simulink model "StateSpaceDynamic"  (R2018a)
settings: Solver=VariableStepAuto  StartTime=0.0  StopTime=10.0  RelTol=1e-3
model workspace (MAT data in the model file):
  Iz = 0.05807429185
  cf = 50000
  cr = 50000
  k1 = 1
  k2 = 0.5673
  k3 = 2.6383
  k4 = 0.4975
  lf = 0.16002
  lr = 0.16002
  m = 2.26796
libraries: cstblocks x1
settings Model: Creator=aswer  LastModifiedBy=aswer

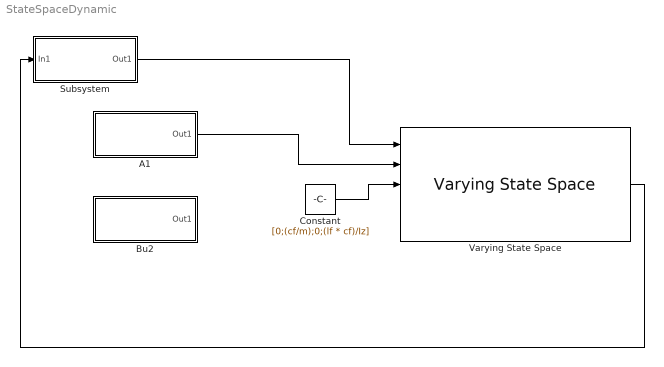
== system StateSpaceDynamic ==
  A1 : Subsystem
  Bu2 : Subsystem
  Constant : Constant  Value=[0;(cf/m);0;(lf * cf)/Iz]  VectorParams1D=off
  Subsystem : Subsystem
  Varying State Space : cstblocks/Linear Parameter Varying/Varying State Space  x0=0  xNames=''  OutputX=on  OutputDX=on
      settings: SourceProductName=Control System Toolbox
  wires:
  Varying State Space/2 -> Subsystem/1(In1)
  A1/1(Out1) -> Varying State Space/2
  Constant/1 -> Varying State Space/3
  Subsystem/1(Out1) -> Varying State Space/1

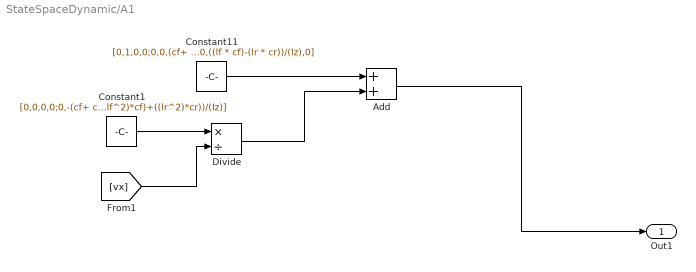
== system StateSpaceDynamic/A1 ==
  Add : Sum
  Constant1 : Constant  Value=[0,0,0,0;0,-(cf+ cr)/(m),0,(lr * cr)-(lf * cf)/(m);0,0,0,0;0,((lr * cr)-(lf * cf))/(Iz),0,-(((lf^2)*cf)+((lr^2)*cr))/(Iz)]  VectorParams1D=off
  Constant11 : Constant  Value=[0,1,0,0;0,0,(cf+ cr)/(m),0;0,0,0,1;0,0,((lf * cf)-(lr * cr))/(Iz),0]  VectorParams1D=off
  Divide : Product  Inputs=*/
  Out1 : Outport
  wires:
  [vx] -> Divide/2
  Constant11/1 -> Add/1
  Constant1/1 -> Divide/1
  Divide/1 -> Add/2
  Add/1 -> Out1/1

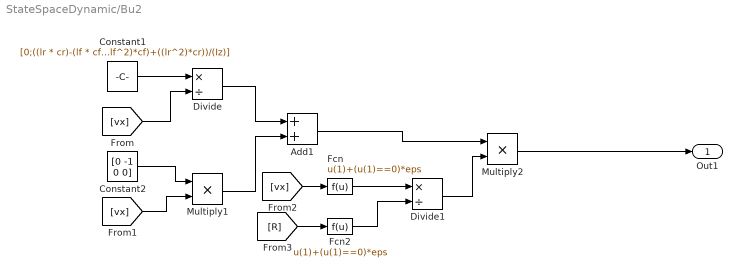
== system StateSpaceDynamic/Bu2 ==
  Add1 : Sum
  Constant1 : Constant  Value=[0;((lr * cr)-(lf * cf))/m;0;-(((lf^2)*cf)+((lr^2)*cr))/(Iz)]  VectorParams1D=off
  Constant2 : Constant  Value=[0 -1 0 0]
  Divide : Product  Inputs=*/
  Divide1 : Product  Inputs=*/
  Fcn : Fcn  Expr=u(1)+(u(1)==0)*eps
  Fcn2 : Fcn  Expr=u(1)+(u(1)==0)*eps
  Multiply1 : Product
  Multiply2 : Product
  Out1 : Outport
  wires:
  Multiply2/1 -> Out1/1
  Constant1/1 -> Divide/1
  [vx] -> Divide/2
  Constant2/1 -> Multiply1/1
  [vx] -> Multiply1/2
  Divide/1 -> Add1/1
  Multiply1/1 -> Add1/2
  Add1/1 -> Multiply2/1
  [vx] -> Fcn/1
  [R] -> Fcn2/1
  Divide1/1 -> Multiply2/2
  Fcn/1 -> Divide1/1
  Fcn2/1 -> Divide1/2

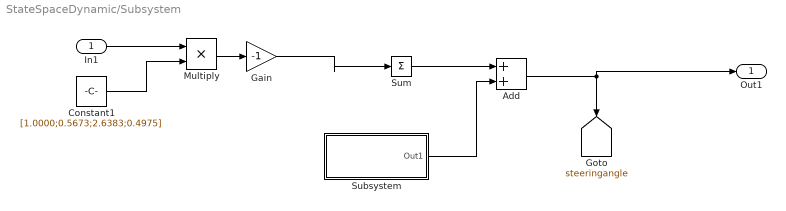
== system StateSpaceDynamic/Subsystem ==
  In1 : Inport
  Add : Sum
  Constant1 : Constant  Value=[1.0000;0.5673;2.6383;0.4975]
  Gain : Gain  Gain=-1
  Multiply : Product
  Subsystem : Subsystem
  Sum : Sum  Inputs=|+
  Out1 : Outport
  tag scope: steeringangle=global
  wires:
  In1/1 -> Multiply/1
  Constant1/1 -> Multiply/2
  Multiply/1 -> Gain/1
  Gain/1 -> Sum/1
  Subsystem/1(Out1) -> Add/2
  Add/1 -> Out1/1, [steeringangle]
  Sum/1 -> Add/1

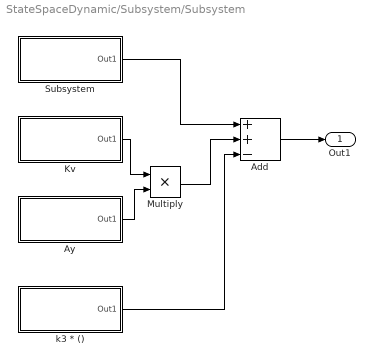
== system StateSpaceDynamic/Subsystem/Subsystem ==
  Add : Sum  Inputs=++-
  Ay : Subsystem
  Kv : Subsystem
  Multiply : Product
  Subsystem : Subsystem
  k3 * () : Subsystem
  Out1 : Outport
  wires:
  Kv/1(Out1) -> Multiply/1
  Ay/1(Out1) -> Multiply/2
  Multiply/1 -> Add/2
  Add/1 -> Out1/1
  k3 * ()/1(Out1) -> Add/3
  Subsystem/1(Out1) -> Add/1

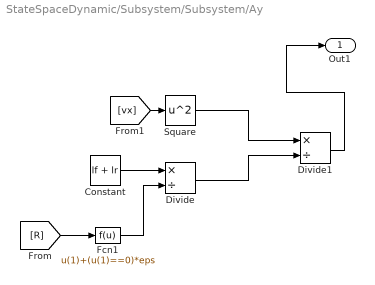
== system StateSpaceDynamic/Subsystem/Subsystem/Ay ==
  Constant : Constant  Value=lf + lr
  Divide : Product  Inputs=*/
  Divide1 : Product  Inputs=*/
  Fcn1 : Fcn  Expr=u(1)+(u(1)==0)*eps
  Square : Math  Operator=square  SaturateOnIntegerOverflow=on
  Out1 : Outport
  wires:
  Constant/1 -> Divide/1
  [R] -> Fcn1/1
  Square/1 -> Divide1/1
  Divide/1 -> Divide1/2
  [vx] -> Square/1
  Divide1/1 -> Out1/1
  Fcn1/1 -> Divide/2

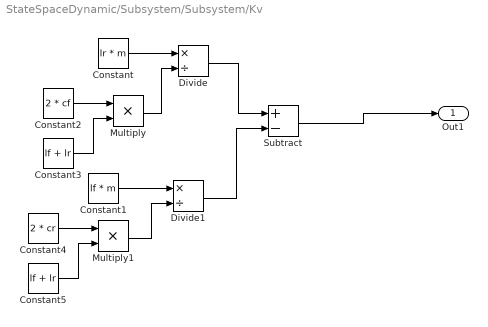
== system StateSpaceDynamic/Subsystem/Subsystem/Kv ==
  Constant : Constant  Value=lr * m
  Constant1 : Constant  Value=lf * m
  Constant2 : Constant  Value=2 * cf
  Constant3 : Constant  Value=lf + lr
  Constant4 : Constant  Value=2 * cr
  Constant5 : Constant  Value=lf + lr
  Divide : Product  Inputs=*/
  Divide1 : Product  Inputs=*/
  Multiply : Product
  Multiply1 : Product
  Subtract : Sum  Inputs=+-
  Out1 : Outport
  wires:
  Divide/1 -> Subtract/1
  Divide1/1 -> Subtract/2
  Constant/1 -> Divide/1
  Constant1/1 -> Divide1/1
  Constant2/1 -> Multiply/1
  Constant3/1 -> Multiply/2
  Multiply/1 -> Divide/2
  Constant5/1 -> Multiply1/2
  Constant4/1 -> Multiply1/1
  Multiply1/1 -> Divide1/2
  Subtract/1 -> Out1/1

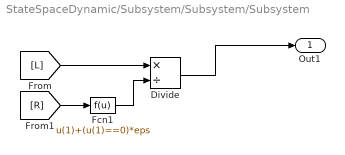
== system StateSpaceDynamic/Subsystem/Subsystem/Subsystem ==
  Divide : Product  Inputs=*/
  Fcn1 : Fcn  Expr=u(1)+(u(1)==0)*eps
  Out1 : Outport
  wires:
  [L] -> Divide/1
  Divide/1 -> Out1/1
  [R] -> Fcn1/1
  Fcn1/1 -> Divide/2

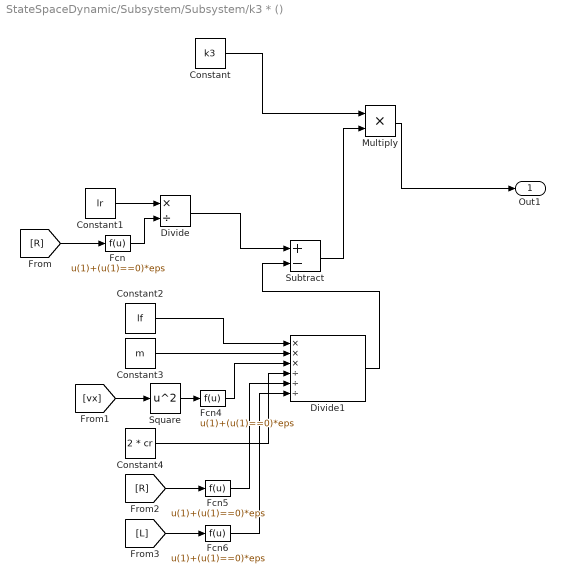
== system StateSpaceDynamic/Subsystem/Subsystem/k3 * () ==
  Constant : Constant  Value=k3
  Constant1 : Constant  Value=lr
  Constant2 : Constant  Value=lf
  Constant3 : Constant  Value=m
  Constant4 : Constant  Value=2 * cr
  Divide : Product  Inputs=*/
  Divide1 : Product  Inputs=***///
  Fcn{,4..6} (4 alike) : Fcn  Expr=u(1)+(u(1)==0)*eps
  Multiply : Product
  Square : Math  Operator=square  SaturateOnIntegerOverflow=on
  Subtract : Sum  Inputs=+-
  Out1 : Outport
  wires:
  Constant/1 -> Multiply/1
  Multiply/1 -> Out1/1
  Divide/1 -> Subtract/1
  Constant1/1 -> Divide/1
  Divide1/1 -> Subtract/2
  Constant2/1 -> Divide1/1
  Constant3/1 -> Divide1/2
  [vx] -> Square/1
  Square/1 -> Fcn4/1
  Constant4/1 -> Divide1/4
  [R] -> Fcn5/1
  [L] -> Fcn6/1
  Subtract/1 -> Multiply/2
  [R] -> Fcn/1
  Fcn6/1 -> Divide1/6
  Fcn5/1 -> Divide1/5
  Fcn4/1 -> Divide1/3
  Fcn/1 -> Divide/2
